simulink model "SpeedController_Module"  (R2025a)
settings: Solver=VariableStepAuto
undefined symbols (not defined in the file): speed_tolerance
libraries: simulink x1
settings Model: Creator=ASUS  LastModifiedBy=ASUS

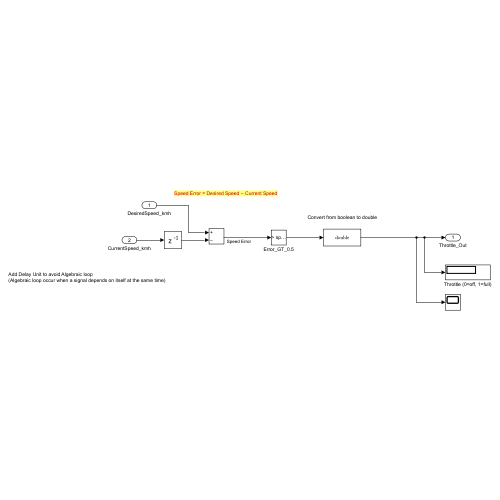
[thumbnail: Simulink's stored preview of the top-level diagram]
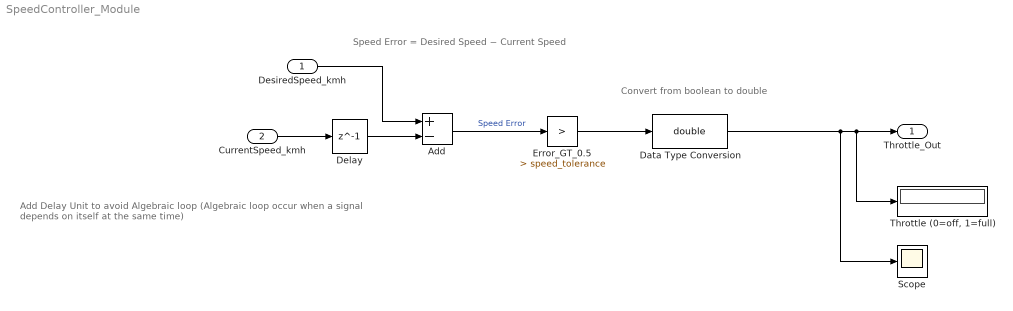
== system SpeedController_Module ==
  note: Add Delay Unit to avoid Algebraic loop
      | (Algebraic loop occur when a signal depends on itself at the same time)
  note: Convert from boolean to double
  note: Speed Error = Desired Speed − Current Speed
  DesiredSpeed_kmh : Inport
  CurrentSpeed_kmh : Inport  Port=2
  Add : Sum  Inputs=+-
  Data Type Conversion : DataTypeConversion  OutDataTypeStr=double  SaturateOnIntegerOverflow=off  RndMeth=Floor
  Delay : Delay  DelayLength=1  InitialCondition=0  SampleTime=0.01
  Error_GT_0.5 : simulink/Logic and Bit Operations/Compare To Constant  relop=>  const=speed_tolerance  OutDataTypeStr=boolean
  Scope : Scope
      settings: ActiveDisplayYMinimum=-0.27595136088709715  ActiveDisplayYMaximum=1.1710798891129031
  "Throttle (0=off, 1=full)" : Display
  Throttle_Out : Outport
  wires:
  DesiredSpeed_kmh/1 -> Add/1
  CurrentSpeed_kmh/1 -> Delay/1
  Add/1 -> Error_GT_0.5/1  "Speed Error"
  Error_GT_0.5/1 -> Data Type Conversion/1
  Data Type Conversion/1 -> Scope/1, "Throttle (0=off, 1=full)"/1, Throttle_Out/1
  Delay/1 -> Add/2
